simulink model "HighPassFilter"  (R2020a)
settings: Solver=FixedStepDiscrete  StartTime=0.0  StopTime=tStop  FixedStep=dt  RelTol=1e-3
settings Model: Creator=Admin  LastModifiedBy=Admin
settings DataIOCC: ExternalInput=[t, noise]  LoadExternalInput=on  SaveFormat=Array  ReturnWorkspaceOutputs=off  TimeSaveName=tfil  OutputSaveName=yfil

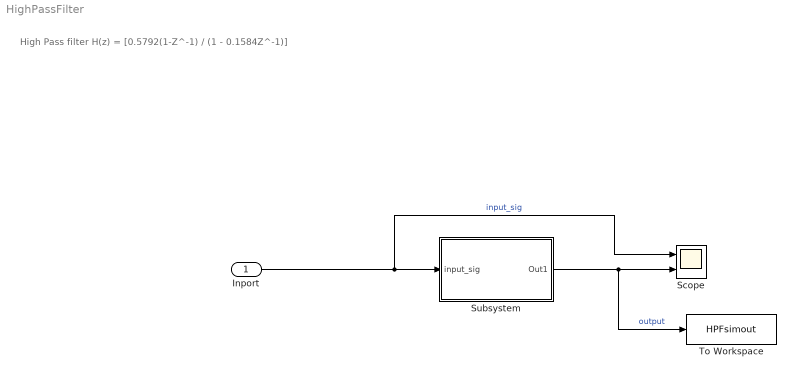
== system HighPassFilter ==
  note: High Pass filter
      |
      | H(z) = [0.5792(1-Z^-1) / (1 - 0.1584Z^-1)]
  Inport : Inport
  Scope : Scope  NumInputPorts=2
  Subsystem : Subsystem  TreatAsAtomicUnit=on
  To Workspace : ToWorkspace  VariableName=HPFsimout  SampleTime=-1
  wires:
  Inport/1 -> Scope/1, Subsystem/1(input_sig)  "input_sig"
  Subsystem/1(Out1) -> To Workspace/1, Scope/2  "output"

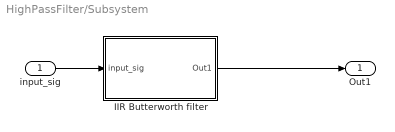
== system HighPassFilter/Subsystem ==
  input_sig : Inport
  IIR Butterworth filter : Subsystem
  Out1 : Outport
  wires:
  IIR Butterworth filter/1(Out1) -> Out1/1
  input_sig/1 -> IIR Butterworth filter/1(input_sig)

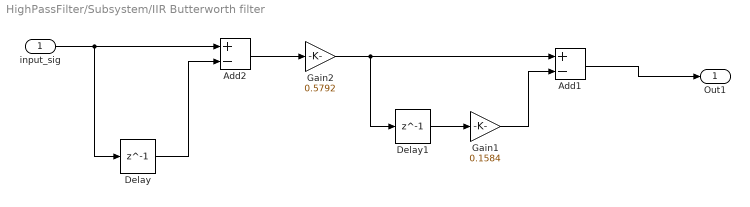
== system HighPassFilter/Subsystem/IIR Butterworth filter ==
  input_sig : Inport
  Add1 : Sum  Inputs=+-
  Add2 : Sum  Inputs=+-
  Delay : Delay  DelayLength=1
  Delay1 : Delay  DelayLength=1
  Gain1 : Gain  Gain=0.1584
  Gain2 : Gain  Gain=0.5792
  Out1 : Outport
  wires:
  input_sig/1 -> Delay/1, Add2/1
  Gain1/1 -> Add1/2
  Gain2/1 -> Add1/1, Delay1/1
  Delay/1 -> Add2/2
  Add1/1 -> Out1/1
  Add2/1 -> Gain2/1
  Delay1/1 -> Gain1/1
